simulink model "Long_Simul_2"  (R2022b)
settings: Solver=VariableStepAuto  StartTime=0.0  StopTime=Inf  RelTol=1e-3
values from neighbouring files (symbols this model uses):
  Af = 4    [ABS_Simul_Initialize.m]    (also in ACC_CTG_Multi_Simul_Initialize.m; ACC_Space_Single_Simul_Initialize.m; ACC_Space_multi_Simul_Initialize.m; CruiseControl_Initialize.m)
  Brake_Input_Amplitude = 5e6*2    (= 10000000)    [ABS_Simul_Initialize.m]    (also in Long_Simul_1_Initialize.m = 100; Long_Simul_2_Initialize.m = 7500000; Long_Simul_3_Initialize.m = 7500000)
  Brake_Input_start_time = 8    [ABS_Simul_Initialize.m]    (also in Long_Simul_1_Initialize.m; Long_Simul_2_Initialize.m; Long_Simul_3_Initialize.m)
  Cd = 0.3    [ABS_Simul_Initialize.m]    (also in ACC_CTG_Multi_Simul_Initialize.m; ACC_Space_Single_Simul_Initialize.m; ACC_Space_multi_Simul_Initialize.m; CruiseControl_Initialize.m)
  g = 9.81    [ABS_Simul_Initialize.m]    (also in ACC_CTG_Multi_Simul_Initialize.m; ACC_Space_Single_Simul_Initialize.m; ACC_Space_multi_Simul_Initialize.m; CruiseControl_Initialize.m)
  m = 1500    [ABS_Simul_Initialize.m]    (also in ACC_CTG_Multi_Simul_Initialize.m; ACC_Space_Single_Simul_Initialize.m; ACC_Space_multi_Simul_Initialize.m; CruiseControl_Initialize.m)
  R_roll = 0.015    [CruiseControl_Initialize.m]    (also in Long_Simul_1_Initialize.m; Long_Simul_2_Initialize.m)
  rho = 1.225    [ABS_Simul_Initialize.m]    (also in ACC_CTG_Multi_Simul_Initialize.m; ACC_Space_Single_Simul_Initialize.m; ACC_Space_multi_Simul_Initialize.m; CruiseControl_Initialize.m)
  Throttle_Input_Amplitude = 30    [ABS_Simul_Initialize.m]    (also in Long_Simul_1_Initialize.m; Long_Simul_2_Initialize.m; Long_Simul_3_Initialize.m)
  Throttle_Input_period = 4    [ABS_Simul_Initialize.m]    (also in Long_Simul_1_Initialize.m; Long_Simul_2_Initialize.m; Long_Simul_3_Initialize.m)
libraries: autolibshared x1
(part 2 of 2)

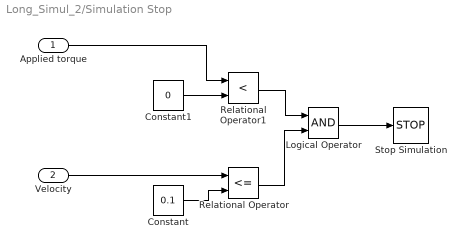
== system Long_Simul_2/Simulation Stop ==
  Applied torque : Inport
  Velocity : Inport  Port=2
  Constant : Constant  Value=0.1
  Constant1 : Constant  Value=0
  Logical Operator : Logic  AllPortsSameDT=off  OutDataTypeStr=boolean
  Relational Operator : RelationalOperator  Operator=<=  OutDataTypeStr=boolean  RndMeth=Simplest  InputSameDT=off
  Relational Operator1 : RelationalOperator  Operator=<  OutDataTypeStr=boolean  RndMeth=Simplest  InputSameDT=off
  Stop Simulation : Stop
  wires:
  Relational Operator1/1 -> Logical Operator/1
  Relational Operator/1 -> Logical Operator/2
  Constant/1 -> Relational Operator/2
  Constant1/1 -> Relational Operator1/2
  Logical Operator/1 -> Stop Simulation/1
  Velocity/1 -> Relational Operator/1
  Applied torque/1 -> Relational Operator1/1

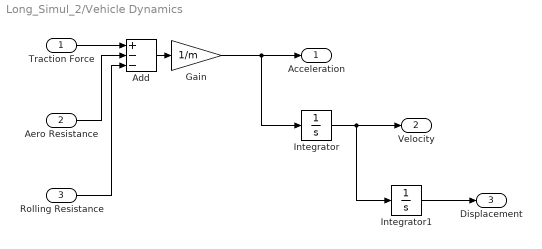
== system Long_Simul_2/Vehicle Dynamics ==
  Traction Force : Inport
  Aero Resistance : Inport  Port=2
  Rolling Resistance : Inport  Port=3
  Add : Sum  Inputs=+--
  Gain : Gain  Gain=1/m
  Integrator : Integrator
  Integrator1 : Integrator
  Acceleration : Outport
  Velocity : Outport  Port=2
  Displacement : Outport  Port=3
  wires:
  Integrator1/1 -> Displacement/1
  Gain/1 -> Integrator/1, Acceleration/1
  Integrator/1 -> Integrator1/1, Velocity/1
  Add/1 -> Gain/1
  Traction Force/1 -> Add/1
  Aero Resistance/1 -> Add/2
  Rolling Resistance/1 -> Add/3

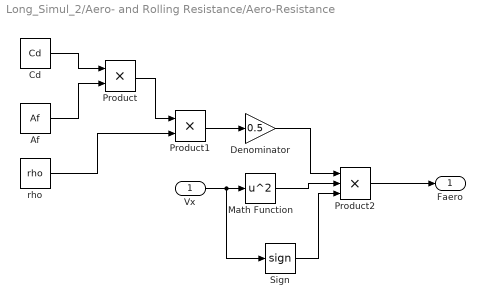
== system Long_Simul_2/Aero- and Rolling Resistance/Aero-Resistance ==
  Vx : Inport
  Af : Constant  Value=Af
  Cd : Constant  Value=Cd
  Denominator : Gain  Gain=0.5
  Math Function : Math  Operator=square  SignedPower=on
  Product : Product
  Product1 : Product
  Product2 : Product  Inputs=3
  Sign : Signum
  rho : Constant  Value=rho
  Faero : Outport  VectorParamsAs1DForOutWhenUnconnected=off
  wires:
  Af/1 -> Product/2
  Product1/1 -> Denominator/1
  Denominator/1 -> Product2/1
  Vx/1 -> Sign/1, Math Function/1
  rho/1 -> Product1/2
  Cd/1 -> Product/1
  Math Function/1 -> Product2/2
  Product/1 -> Product1/1
  Sign/1 -> Product2/3
  Product2/1 -> Faero/1

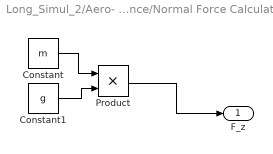
== system Long_Simul_2/Aero- and Rolling Resistance/Normal Force Calculation ==
  Constant : Constant  Value=m
  Constant1 : Constant  Value=g
  Product : Product
  F_z : Outport
  wires:
  Product/1 -> F_z/1
  Constant1/1 -> Product/2
  Constant/1 -> Product/1

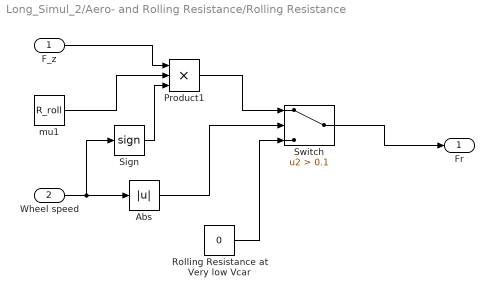
== system Long_Simul_2/Aero- and Rolling Resistance/Rolling Resistance ==
  F_z : Inport
  Wheel speed : Inport  Port=2
  Abs : Abs  SaturateOnIntegerOverflow=off
  Product1 : Product  Inputs=3
  Rolling Resistance at Very low Vcar : Constant  Value=0
  Sign : Signum
  Switch : Switch  Criteria=u2 > Threshold  Threshold=0.1  SaturateOnIntegerOverflow=off  InputSameDT=off
  mu1 : Constant  Value=R_roll
  Fr : Outport  VectorParamsAs1DForOutWhenUnconnected=off
  wires:
  F_z/1 -> Product1/1
  Product1/1 -> Switch/1
  Rolling Resistance at Very low Vcar/1 -> Switch/3
  mu1/1 -> Product1/2
  Wheel speed/1 -> Sign/1, Abs/1
  Abs/1 -> Switch/2
  Sign/1 -> Product1/3
  Switch/1 -> Fr/1

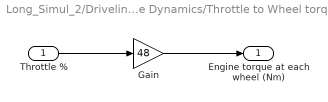
== system Long_Simul_2/Driveline Dynamics/Throttle to Wheel torque ==
  Throttle % : Inport
  Gain : Gain  Gain=48
  Engine torque at each wheel (Nm) : Outport  VectorParamsAs1DForOutWhenUnconnected=off
  wires:
  Throttle %/1 -> Gain/1
  Gain/1 -> Engine torque at each wheel (Nm)/1
